simulink model "bicyclemodel_step_disturbance_force"  (R2021a)
settings: Solver=FixedStepAuto  StartTime=0.0  StopTime=tf  FixedStep=dt  RelTol=1e-3
values from neighbouring files (symbols this model uses):
  I = 2500    [E4_1.m]
  Kf = 55000    [E4_1.m]
  Kr = 60000    [E4_1.m]
  lf = 1.1    [E4_1.m]
  lr = 1.6    [E4_1.m]
  m = 1500    [E4_1.m]
  Sf = 0.0    (= 0)    [E4_1.m]
  V = 80/3.6    (= 22.2222222222)    [E4_1.m]
  Y0 = 4000    [E4_1.m]
libraries: simulink x1
settings Model: Creator=abeam  LastModifiedBy=abeam

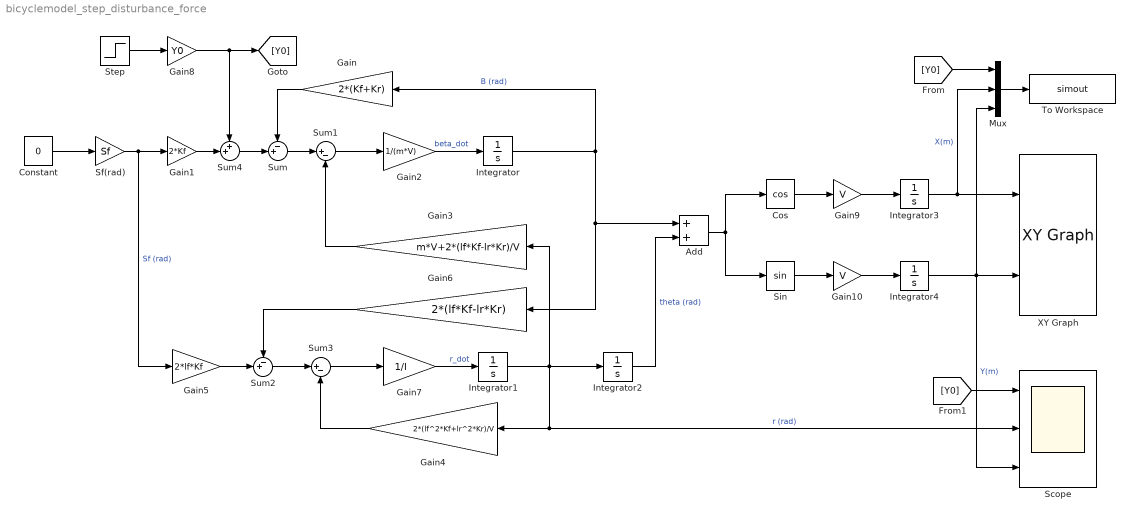
== system bicyclemodel_step_disturbance_force ==
  Add : Sum
  Constant : Constant  Value=0
  Cos : Trigonometry  Operator=cos
  Gain : Gain  Gain=2*(Kf+Kr)
  Gain1 : Gain  Gain=2*Kf
  Gain10 : Gain  Gain=V
  Gain2 : Gain  Gain=1/(m*V)
  Gain3 : Gain  Gain=m*V+2*(lf*Kf-lr*Kr)/V
  Gain4 : Gain  Gain=2*(lf^2*Kf+lr^2*Kr)/V
  Gain5 : Gain  Gain=2*lf*Kf
  Gain6 : Gain  Gain=2*(lf*Kf-lr*Kr)
  Gain7 : Gain  Gain=1/I
  Gain8 : Gain  Gain=Y0
  Gain9 : Gain  Gain=V
  Integrator{,1..4} (5 alike) : Integrator
  Mux : Mux  Inputs=3
  Scope : Scope  NumInputPorts=3
  Sf(rad) : Gain  Gain=Sf
  Sin : Trigonometry
  Step : Step  SampleTime=0
  Sum : Sum  Inputs=-+|
  Sum1 : Sum  Inputs=|+-
  Sum2 : Sum  Inputs=-+|
  Sum3 : Sum  Inputs=|+-
  Sum4 : Sum  Inputs=++|
  To Workspace : ToWorkspace  VariableName=simout  SaveFormat=Timeseries  SampleTime=-1
  XY Graph : simulink/Sinks/XY Graph  xmin=0  xmax=80  ymin=-5  ymax=5  st=-1
  wires:
  Constant/1 -> Sf(rad)/1
  Sf(rad)/1 -> Gain5/1, Gain1/1  "Sf (rad)"
  Sum/1 -> Sum1/1
  Gain/1 -> Sum/1
  Sum1/1 -> Gain2/1
  Gain2/1 -> Integrator/1  "beta_dot"
  Integrator/1 -> Add/1, Gain6/1, Gain/1  "B (rad)"
  Gain3/1 -> Sum1/2
  Gain5/1 -> Sum2/2
  Sum2/1 -> Sum3/1
  Gain6/1 -> Sum2/1
  Sum3/1 -> Gain7/1
  Gain4/1 -> Sum3/2
  Gain7/1 -> Integrator1/1  "r_dot"
  Integrator1/1 -> Gain4/1, Scope/2, Integrator2/1, Gain3/1  "r (rad)"
  Step/1 -> Gain8/1
  Gain1/1 -> Sum4/2
  Sum4/1 -> Sum/2
  Gain8/1 -> Sum4/1, [Y0]
  Integrator2/1 -> Add/2  "theta (rad)"
  Add/1 -> Cos/1, Sin/1
  Cos/1 -> Gain9/1
  Sin/1 -> Gain10/1
  Gain9/1 -> Integrator3/1
  Gain10/1 -> Integrator4/1
  Integrator3/1 -> Mux/2, XY Graph/1  "X(m)"
  Integrator4/1 -> XY Graph/2, Scope/3, Mux/3  "Y(m)"
  [Y0] -> Mux/1
  Mux/1 -> To Workspace/1
  [Y0] -> Scope/1
